simulink model "DC_motor_response"  (R2016a)
settings: Solver=VariableStepAuto  StartTime=0.0  StopTime=10.0  FixedStep=0.001  RelTol=1e-3
settings Model: Creator=mgreiff  LastModifiedBy=mgreiff
settings DataIOCC: LimitDataPoints=on
settings DebuggingCC: AllowSymbolicDim=off
settings ModelReferenceCC: PropagateSignalLabelsOutOfModel=off
settings GRTTargetCC: GeneratePreprocessorConditionals=Use local settings

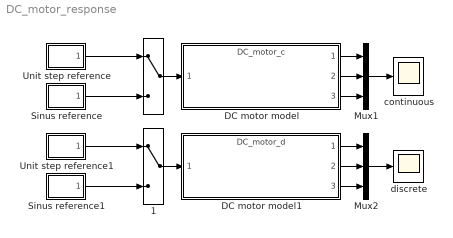
== system DC_motor_response ==
  "   " : ManualSwitch
  "   1" : ManualSwitch
  DC motor model : ModelReference  ModelNameDialog=DC_motor_c.slx  SimulationMode=Normal  ModelReferenceVersion=1.8
  DC motor model1 : ModelReference  ModelNameDialog=DC_motor_d.slx  SimulationMode=Normal  ModelReferenceVersion=1.8
  Mux1 : Mux  Inputs=3
  Mux2 : Mux  Inputs=3
  Sinus reference : Subsystem
  Sinus reference1 : Subsystem
  Unit step reference : Subsystem
  Unit step reference1 : Subsystem
  continuous : Scope
  discrete : Scope
  wires:
  "   "/1 -> DC motor model/1
  Unit step reference/1(voltage) -> "   "/1
  Sinus reference/1(voltage) -> "   "/2
  "   1"/1 -> DC motor model1/1
  Unit step reference1/1(voltage) -> "   1"/1
  Sinus reference1/1(voltage) -> "   1"/2
  DC motor model1/1 -> Mux2/1
  DC motor model1/2 -> Mux2/2
  DC motor model1/3 -> Mux2/3
  DC motor model/1 -> Mux1/1
  DC motor model/2 -> Mux1/2
  DC motor model/3 -> Mux1/3
  Mux2/1 -> discrete/1
  Mux1/1 -> continuous/1

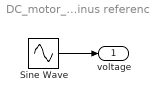
== system DC_motor_response/Sinus reference ==
  Sine Wave : Sin  SampleTime=0
  voltage : Outport
  wires:
  Sine Wave/1 -> voltage/1

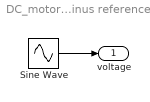
== system DC_motor_response/Sinus reference1 ==
  Sine Wave : Sin  SampleTime=0
  voltage : Outport
  wires:
  Sine Wave/1 -> voltage/1

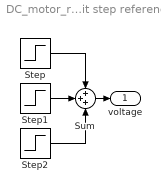
== system DC_motor_response/Unit step reference ==
  Step : Step  Time=0  SampleTime=0
  Step1 : Step  Time=4  After=-2  SampleTime=0
  Step2 : Step  Time=8  SampleTime=0
  Sum : Sum  Inputs=+++
  voltage : Outport
  wires:
  Sum/1 -> voltage/1
  Step1/1 -> Sum/2
  Step2/1 -> Sum/3
  Step/1 -> Sum/1

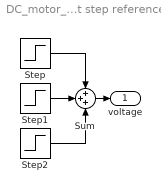
== system DC_motor_response/Unit step reference1 ==
  Step : Step  Time=0  SampleTime=0
  Step1 : Step  Time=4  After=-2  SampleTime=0
  Step2 : Step  Time=8  SampleTime=0
  Sum : Sum  Inputs=+++
  voltage : Outport
  wires:
  Sum/1 -> voltage/1
  Step1/1 -> Sum/2
  Step2/1 -> Sum/3
  Step/1 -> Sum/1
